simulink model "IC_Project"  (R2022b)
settings: Solver=FixedStepAuto  StartTime=0.0  StopTime=50  FixedStep=Ts  RelTol=1e-6
values from neighbouring files (symbols this model uses):
  g = 9.81    [aero_guid_dat.m]
  Iyy = 182.5/(Kg2slug*m2ft^2)    (= 247.436636441)    [aero_guid_dat.m]
  R = 287.26    [aero_guid_dat.m]
undefined symbols (not defined in the file or in its folder): AF, b_u, Delta_u, Delta_z_rotor, Dis, E_a, GE_flag, I_rotor, IC, inertia_u, Ixx, Izz, K1, K2, K3, K4, k_e, k_m, lambda, m, m_u, N_n, N_p, N_u, n_u, n_y, Out_sampleTime, phi_max, Q, R_eq, T_M, T_u, T_u_u, tau_m, theta_max, Ts
libraries: sharedtransform x1, sharedutil x1, simulink x1
settings Model: Creator=Mahdi  LastModifiedBy=Mahdi

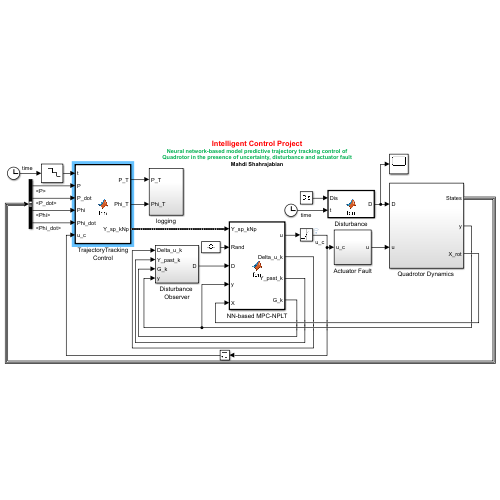
[thumbnail: Simulink's stored preview of the top-level diagram]
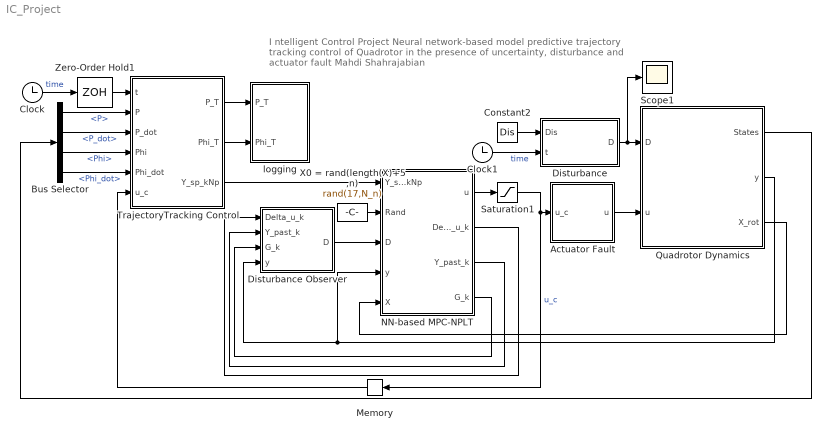
== system IC_Project ==
  note: I ntelligent Control Project
      | Neural network-based model predictive trajectory tracking control of Quadrotor in the presence of uncertainty, disturbance and actuator fault
      | Mahdi Shahrajabian
  Actuator Fault : Subsystem
  Bus Selector : BusSelector  OutputSignals=P,P_dot,Phi,Phi_dot
  Clock : Clock
  Clock1 : Clock
  Constant2 : Constant  Value=Dis
  Disturbance : MATLAB Function  TreatAsAtomicUnit=on
  Disturbance Observer : Subsystem
  Memory : Memory  InitialCondition=m*g*[1;1;1;1]/4
  NN-based MPC-NPLT : MATLAB Function  TreatAsAtomicUnit=on
  "Quadrotor Dynamics " : Subsystem  VariantControl=Choice_1
  Saturation1 : Saturate  UpperLimit=T_M  LowerLimit=0
  Scope1 : Scope
  TrajectoryTracking Control : MATLAB Function  TreatAsAtomicUnit=on
  X0 = rand(length(X)+5,n) : Constant  Value=rand(17,N_n)
  Zero-Order Hold1 : ZeroOrderHold  SampleTime=Ts
  logging : Subsystem
  wires:
  "Quadrotor Dynamics "/3(X_rot) -> NN-based MPC-NPLT/5(X)
  Zero-Order Hold1/1 -> TrajectoryTracking Control/1(t)
  Memory/1 -> TrajectoryTracking Control/6(u_c)
  "Quadrotor Dynamics "/1(States) -> Bus Selector/1
  Clock/1 -> Zero-Order Hold1/1  "time"
  Bus Selector/1 -> TrajectoryTracking Control/2(P)  "<P>"
  Bus Selector/2 -> TrajectoryTracking Control/3(P_dot)  "<P_dot>"
  Bus Selector/3 -> TrajectoryTracking Control/4(Phi)  "<Phi>"
  Bus Selector/4 -> TrajectoryTracking Control/5(Phi_dot)  "<Phi_dot>"
  TrajectoryTracking Control/3(Y_sp_kNp) -> NN-based MPC-NPLT/1(Y_sp_kNp)
  Disturbance/1(D) -> Scope1/1, "Quadrotor Dynamics "/1(D)
  TrajectoryTracking Control/2(Phi_T) -> logging/2(Phi_T)
  TrajectoryTracking Control/1(P_T) -> logging/1(P_T)
  X0 = rand(length(X)+5,n)/1 -> NN-based MPC-NPLT/2(Rand)
  "Quadrotor Dynamics "/2(y) -> NN-based MPC-NPLT/4(y), Disturbance Observer/4(y)
  Disturbance Observer/1(D) -> NN-based MPC-NPLT/3(D)
  NN-based MPC-NPLT/2(Delta_u_k) -> Disturbance Observer/1(Delta_u_k)
  NN-based MPC-NPLT/3(Y_past_k) -> Disturbance Observer/2(Y_past_k)
  NN-based MPC-NPLT/4(G_k) -> Disturbance Observer/3(G_k)
  Constant2/1 -> Disturbance/1(Dis)
  Actuator Fault/1(u) -> "Quadrotor Dynamics "/2(u)
  Clock1/1 -> Disturbance/2(t)  "time"
  NN-based MPC-NPLT/1(u) -> Saturation1/1
  Saturation1/1 -> Memory/1, Actuator Fault/1(u_c)  "u_c"

== system IC_Project/Actuator Fault ==
  u_c : Inport
  Actuator Fault1 : MATLAB Function  TreatAsAtomicUnit=on
  Clock : Clock
  Constant3 : Constant  Value=AF
  Scope : Scope
  Zero-Order Hold : ZeroOrderHold  SampleTime=Ts
  u : Outport
  wires:
  Zero-Order Hold/1 -> Actuator Fault1/2(u_c)
  Constant3/1 -> Actuator Fault1/1(AF)
  Clock/1 -> Actuator Fault1/3(t)
  Actuator Fault1/1(u) -> u/1
  u_c/1 -> Zero-Order Hold/1, Scope/1

== system IC_Project/Disturbance Observer ==
  Delta_u_k : Inport
  Y_past_k : Inport  Port=2
  G_k : Inport  Port=3
  y : Inport  Port=4
  MATLAB Function : MATLAB Function  TreatAsAtomicUnit=on
  Previous Steps : Subsystem
  Previous Steps1 : Subsystem
  Previous Steps2 : Subsystem
  D : Outport
  wires:
  MATLAB Function/1(D) -> D/1
  y/1 -> MATLAB Function/1(y)
  Delta_u_k/1 -> Previous Steps/1(Delta_u_k)
  Previous Steps/1(Delta_u_past) -> MATLAB Function/4(Delta_u_past)
  Previous Steps1/1(G_past) -> MATLAB Function/3(G_past)
  Previous Steps2/1(Y_past_past) -> MATLAB Function/2(Y_past_past)
  Y_past_k/1 -> Previous Steps2/1(Y_past_k)
  G_k/1 -> Previous Steps1/1(G_k)

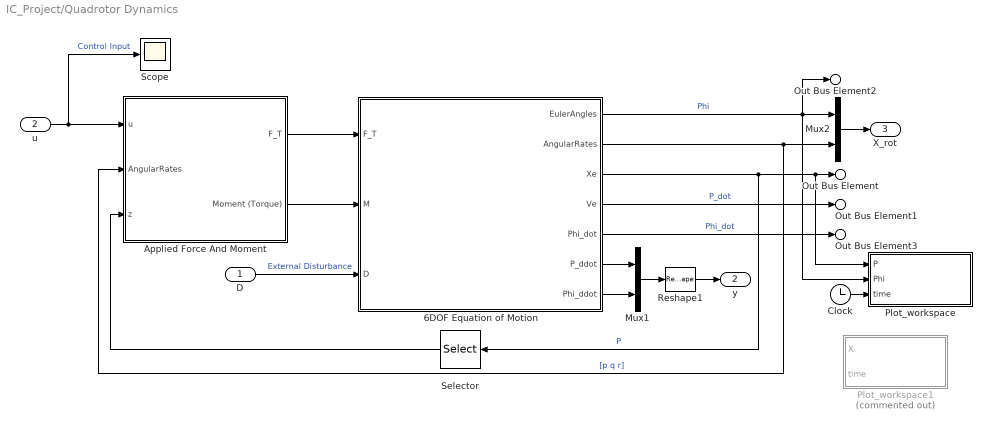
== system IC_Project/Quadrotor Dynamics  ==
  D : Inport
  u : Inport  Port=2
  6DOF Equation of Motion : Subsystem  mask{m=m_u, I=inertia_u, X0=IC.X, V0=IC.V, EA0=IC.EA, RR0=IC.AR}
      mask prompts: m "Quadrotor mass (m) - (kg):"; I "Quadrotor Moment of Inertia matrix (I) - (kg.m^2):"; X0 "Initial position in inertial axes [Xe, Ye, Ze] - (m):"; V0 "Initial velocity in body axes [u,v,w] - (m/s):"; EA0 "Initial Euler angles [roll, pitch, yaw] - (rad):"; RR0 "Initial body rotation rates [p,q,r] - (rad/s):"
      mask help: 6dof equations of motion of quadrotor
      mask DialogControl Container5 Prompt: Parameters
      mask DialogControl Container7 Prompt: Initial conditions
      mask Display: disp("6DOF Equation of motion\n(Euler Angles)")
  Applied Force And Moment : Subsystem  mask{T_u=T_u_u, b=b_u}
  Clock : Clock
  Mux1 : Mux  Inputs=2
  Mux2 : Mux  Inputs=2
  Plot_workspace : Subsystem
  Plot_workspace1 : Subsystem  Commented=on
  Reshape1 : Reshape  OutputDimensionality=Column vector (2-D)
  Scope : Scope
  Selector : Selector  InputPortWidth=3  IndexOptions=Index vector (dialog)  Indices=3  OutputSizes=1
  Out Bus Element : Outport  PortName=States  Element=P
  Out Bus Element1 : Outport  PortName=States  Element=P_dot
  Out Bus Element2 : Outport  PortName=States  Element=Phi
  Out Bus Element3 : Outport  PortName=States  Element=Phi_dot
  y : Outport  Port=2
  X_rot : Outport  Port=3
  wires:
  D/1 -> 6DOF Equation of Motion/3(D)  "External Disturbance"
  u/1 -> Scope/1, Applied Force And Moment/1(u)  "Control Input"
  Applied Force And Moment/2(Moment (Torque)) -> 6DOF Equation of Motion/2(M)
  6DOF Equation of Motion/2(AngularRates) -> Applied Force And Moment/2(AngularRates), Mux2/2  "[p q r]"
  Applied Force And Moment/1(F_T) -> 6DOF Equation of Motion/1(" F_T")
  6DOF Equation of Motion/4(Ve) -> Out Bus Element1/1  "P_dot"
  Selector/1 -> Applied Force And Moment/3(z)
  6DOF Equation of Motion/7(Phi_ddot) -> Mux1/2
  Reshape1/1 -> y/1
  Mux1/1 -> Reshape1/1
  6DOF Equation of Motion/6(P_ddot) -> Mux1/1
  Mux2/1 -> X_rot/1
  6DOF Equation of Motion/3(Xe) -> Selector/1, Plot_workspace/1(P), Out Bus Element/1  "P"
  6DOF Equation of Motion/1(EulerAngles) -> Out Bus Element2/1, Plot_workspace/2(Phi), Mux2/1  "Phi"
  6DOF Equation of Motion/5(Phi_dot) -> Out Bus Element3/1  "Phi_dot"
  Clock/1 -> Plot_workspace/3(time)

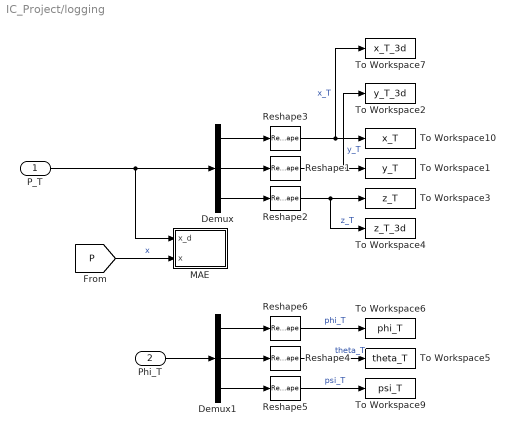
== system IC_Project/logging ==
  P_T : Inport
  Phi_T : Inport  Port=2
  Demux : Demux  Outputs=3
  Demux1 : Demux  Outputs=3
  MAE : Subsystem
  Reshape{1..6} (6 alike) : Reshape
  To Workspace1 : ToWorkspace  VariableName=y_T  SampleTime=Out_sampleTime
  To Workspace10 : ToWorkspace  VariableName=x_T  SampleTime=Out_sampleTime
  To Workspace2 : ToWorkspace  VariableName=y_T_3d  SampleTime=8*Out_sampleTime
  To Workspace3 : ToWorkspace  VariableName=z_T  SampleTime=Out_sampleTime
  To Workspace4 : ToWorkspace  VariableName=z_T_3d  SampleTime=8*Out_sampleTime
  To Workspace5 : ToWorkspace  VariableName=theta_T  SampleTime=Out_sampleTime
  To Workspace6 : ToWorkspace  VariableName=phi_T  SampleTime=Out_sampleTime
  To Workspace7 : ToWorkspace  VariableName=x_T_3d  SampleTime=8*Out_sampleTime
  To Workspace9 : ToWorkspace  VariableName=psi_T  SampleTime=Out_sampleTime
  wires:
  Reshape3/1 -> To Workspace7/1, To Workspace10/1  "x_T"
  Demux/1 -> Reshape3/1
  Demux/3 -> Reshape2/1
  Reshape2/1 -> To Workspace3/1, To Workspace4/1  "z_T"
  Reshape1/1 -> To Workspace2/1, To Workspace1/1  "y_T"
  Demux/2 -> Reshape1/1
  Reshape5/1 -> To Workspace9/1  "psi_T"
  Reshape4/1 -> To Workspace5/1  "theta_T"
  Demux1/2 -> Reshape4/1
  Demux1/1 -> Reshape6/1
  Demux1/3 -> Reshape5/1
  Reshape6/1 -> To Workspace6/1  "phi_T"
  Phi_T/1 -> Demux1/1
  P_T/1 -> Demux/1, MAE/1(x_d)
  [P] -> MAE/2(x)  "x"

== system IC_Project/Disturbance Observer/Previous Steps ==
  Delta_u_k : Inport
  Matrix Concatenate : Concatenate  NumInputs=10  ConcatenateDimension=2
  Reshape : Reshape  OutputDimensionality=Customize  OutputDimensions=[n_u 10]
  Unit Delay{,1..9} (10 alike) : UnitDelay  SampleTime=-1  HasFrameUpgradeWarning=on
  Delta_u_past : Outport
  wires:
  Matrix Concatenate/1 -> Reshape/1
  Delta_u_k/1 -> Unit Delay/1
  Unit Delay/1 -> Matrix Concatenate/1, Unit Delay1/1  "Delta_u_k1"
  Unit Delay1/1 -> Matrix Concatenate/2, Unit Delay2/1  "Delta_u_k2"
  Unit Delay2/1 -> Matrix Concatenate/3, Unit Delay3/1  "Delta_u_k3"
  Unit Delay3/1 -> Matrix Concatenate/4, Unit Delay4/1  "Delta_u_k4"
  Unit Delay4/1 -> Matrix Concatenate/5, Unit Delay5/1  "Delta_u_k5"
  Unit Delay5/1 -> Matrix Concatenate/6, Unit Delay6/1  "Delta_u_k6"
  Unit Delay6/1 -> Matrix Concatenate/7, Unit Delay7/1  "Delta_u_k7"
  Unit Delay7/1 -> Matrix Concatenate/8, Unit Delay8/1  "Delta_u_k8"
  Unit Delay8/1 -> Matrix Concatenate/9, Unit Delay9/1  "Delta_u_k9"
  Unit Delay9/1 -> Matrix Concatenate/10  "Delta_u_k10"
  Reshape/1 -> Delta_u_past/1

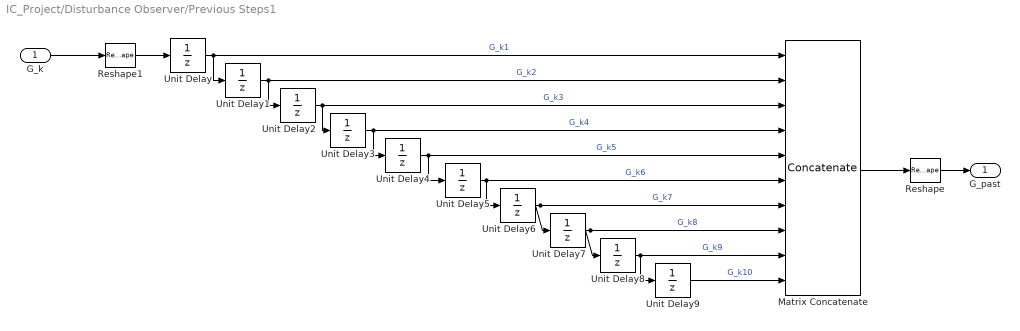
== system IC_Project/Disturbance Observer/Previous Steps1 ==
  G_k : Inport
  Matrix Concatenate : Concatenate  NumInputs=10  Mode=Multidimensional array  ConcatenateDimension=2
  Reshape : Reshape  OutputDimensionality=Customize  OutputDimensions=[60 24 10]
  Reshape1 : Reshape  OutputDimensionality=Customize  OutputDimensions=[60*24 1]
  Unit Delay{,1..9} (10 alike) : UnitDelay  SampleTime=-1  HasFrameUpgradeWarning=on
  G_past : Outport
  wires:
  Unit Delay9/1 -> Matrix Concatenate/10  "G_k10"
  Unit Delay8/1 -> Matrix Concatenate/9, Unit Delay9/1  "G_k9"
  Unit Delay7/1 -> Matrix Concatenate/8, Unit Delay8/1  "G_k8"
  Unit Delay6/1 -> Matrix Concatenate/7, Unit Delay7/1  "G_k7"
  Unit Delay5/1 -> Matrix Concatenate/6, Unit Delay6/1  "G_k6"
  Unit Delay4/1 -> Matrix Concatenate/5, Unit Delay5/1  "G_k5"
  Unit Delay3/1 -> Matrix Concatenate/4, Unit Delay4/1  "G_k4"
  Unit Delay2/1 -> Matrix Concatenate/3, Unit Delay3/1  "G_k3"
  Unit Delay1/1 -> Matrix Concatenate/2, Unit Delay2/1  "G_k2"
  Unit Delay/1 -> Matrix Concatenate/1, Unit Delay1/1  "G_k1"
  G_k/1 -> Reshape1/1
  Matrix Concatenate/1 -> Reshape/1
  Reshape/1 -> G_past/1
  Reshape1/1 -> Unit Delay/1

== system IC_Project/Disturbance Observer/Previous Steps2 ==
  Y_past_k : Inport
  Matrix Concatenate : Concatenate  NumInputs=10  Mode=Multidimensional array  ConcatenateDimension=2
  Reshape : Reshape  OutputDimensionality=Customize  OutputDimensions=[N_p*n_y 10]
  Unit Delay{,1..9} (10 alike) : UnitDelay  SampleTime=-1  HasFrameUpgradeWarning=on
  Y_past_past : Outport
  wires:
  Matrix Concatenate/1 -> Reshape/1
  Y_past_k/1 -> Unit Delay/1
  Unit Delay/1 -> Matrix Concatenate/1, Unit Delay1/1  "Y_past_k1"
  Unit Delay1/1 -> Matrix Concatenate/2, Unit Delay2/1  "Y_past_k2"
  Unit Delay2/1 -> Matrix Concatenate/3, Unit Delay3/1  "Y_past_k3"
  Unit Delay3/1 -> Matrix Concatenate/4, Unit Delay4/1  "Y_past_k4"
  Unit Delay4/1 -> Matrix Concatenate/5, Unit Delay5/1  "Y_past_k5"
  Unit Delay5/1 -> Matrix Concatenate/6, Unit Delay6/1  "Y_past_k6"
  Unit Delay6/1 -> Matrix Concatenate/7, Unit Delay7/1  "Y_past_k7"
  Unit Delay7/1 -> Matrix Concatenate/8, Unit Delay8/1  "Y_past_k8"
  Unit Delay8/1 -> Matrix Concatenate/9, Unit Delay9/1  "Y_past_k9"
  Unit Delay9/1 -> Matrix Concatenate/10  "Y_past_k10"
  Reshape/1 -> Y_past_past/1

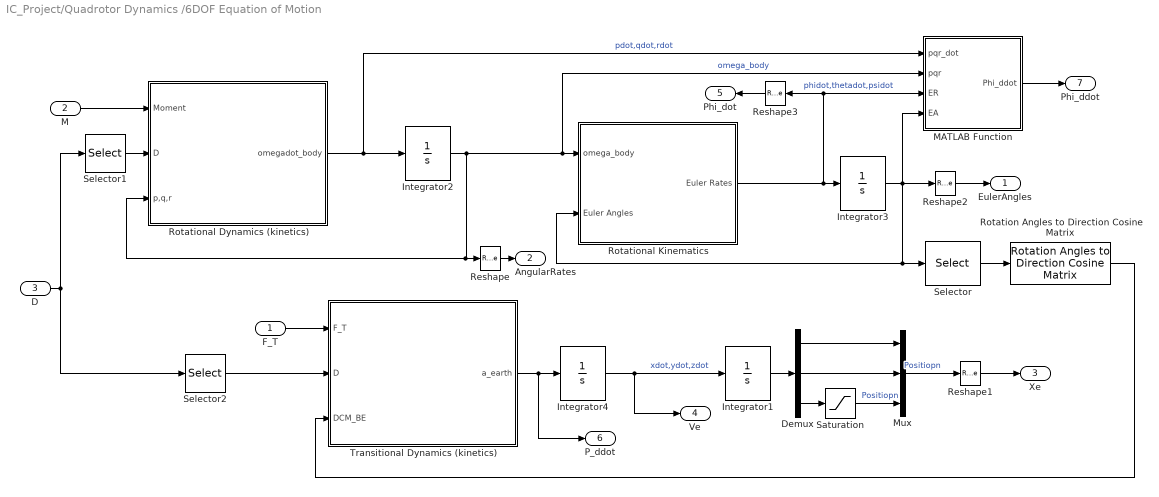
== system IC_Project/Quadrotor Dynamics /6DOF Equation of Motion ==
  " F_T" : Inport
  M : Inport  Port=2
  D : Inport  Port=3
  Demux : Demux  Outputs=3
  Integrator1 : Integrator  InitialCondition=X0
  Integrator2 : Integrator  InitialCondition=RR0
  Integrator3 : Integrator  InitialCondition=EA0  WrapState=on
  Integrator4 : Integrator  InitialCondition=V0
  MATLAB Function : MATLAB Function  TreatAsAtomicUnit=on
  Mux : Mux  Inputs=3
  Reshape{,1..3} (4 alike) : Reshape  OutputDimensionality=Column vector (2-D)
  Rotation Angles to Direction Cosine Matrix : sharedtransform/Rotation Angles to Direction Cosine Matrix  rotationOrder=ZYX  aMode=aMode
  Rotational Dynamics (kinetics) : Subsystem
  Rotational Kinematics : Subsystem
  Saturation : Saturate  UpperLimit=0  LowerLimit=-inf
  Selector : Selector  InputPortWidth=3  IndexOptions=Index vector (dialog)  Indices=[3 2 1]  OutputSizes=1
  Selector1 : Selector  InputPortWidth=6  IndexOptions=Index vector (dialog)  Indices=[1 2 3]  OutputSizes=1
  Selector2 : Selector  InputPortWidth=6  IndexOptions=Index vector (dialog)  Indices=[4 5 6]  OutputSizes=1
  Transitional Dynamics (kinetics) : Subsystem
  EulerAngles : Outport
  AngularRates : Outport  Port=2
  Xe : Outport  Port=3
  Ve : Outport  Port=4
  Phi_dot : Outport  Port=5
  P_ddot : Outport  Port=6
  Phi_ddot : Outport  Port=7
  wires:
  Mux/1 -> Reshape1/1  "Positiopn"
  M/1 -> Rotational Dynamics (kinetics)/1(Moment)
  " F_T"/1 -> Transitional Dynamics (kinetics)/1(" F_T")
  Rotational Kinematics/1(Euler Rates) -> Reshape3/1, MATLAB Function/3(ER), Integrator3/1  "phidot,thetadot,psidot"
  Integrator4/1 -> Ve/1, Integrator1/1  "xdot,ydot,zdot"
  Integrator2/1 -> MATLAB Function/2(pqr), Rotational Kinematics/1(omega_body), Reshape/1, Rotational Dynamics (kinetics)/3(p,q,r)  "omega_body"
  Selector/1 -> Rotation Angles to Direction Cosine Matrix/1
  Integrator3/1 -> MATLAB Function/4(EA), Selector/1, Rotational Kinematics/2(Euler Angles), Reshape2/1
  Rotation Angles to Direction Cosine Matrix/1 -> Transitional Dynamics (kinetics)/3(DCM_BE)
  Transitional Dynamics (kinetics)/1(a_earth) -> P_ddot/1, Integrator4/1
  D/1 -> Selector2/1, Selector1/1
  Selector1/1 -> Rotational Dynamics (kinetics)/2(D)
  Selector2/1 -> Transitional Dynamics (kinetics)/2(D)
  Integrator1/1 -> Demux/1
  Demux/1 -> Mux/1
  Demux/2 -> Mux/2
  Demux/3 -> Saturation/1
  Saturation/1 -> Mux/3  "Positiopn"
  MATLAB Function/1(Phi_ddot) -> Phi_ddot/1
  Rotational Dynamics (kinetics)/1(omegadot_body) -> MATLAB Function/1(pqr_dot), Integrator2/1  "pdot,qdot,rdot"
  Reshape2/1 -> EulerAngles/1
  Reshape1/1 -> Xe/1
  Reshape/1 -> AngularRates/1
  Reshape3/1 -> Phi_dot/1

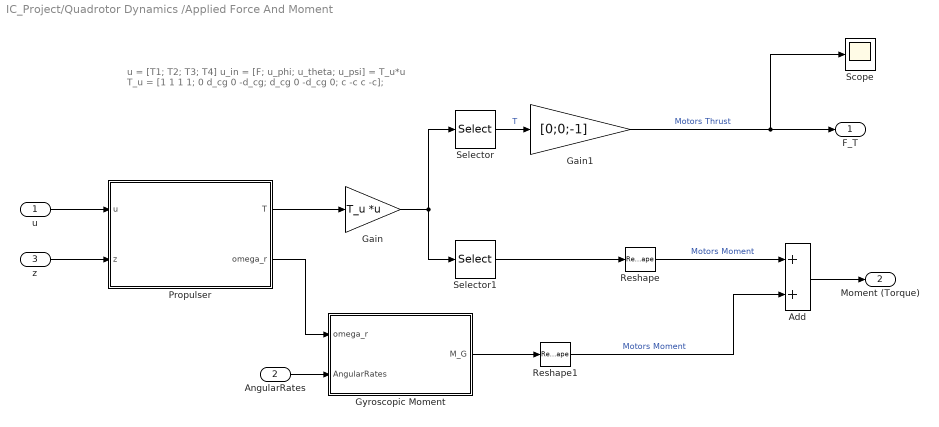
== system IC_Project/Quadrotor Dynamics /Applied Force And Moment ==
  note: u = [T1; T2; T3; T4]
      | u_in = [F; u_phi; u_theta; u_psi] = T_u*u
      | T_u = [1 1 1 1;
      |            0 d_cg 0 -d_cg;
      |           d_cg 0 -d_cg 0;
      |           c -c c -c];
  u : Inport
  AngularRates : Inport  Port=2
  z : Inport  Port=3
  Add : Sum
  Gain : Gain  Gain=T_u  Multiplication=Matrix(K*u)
  Gain1 : Gain  Gain=[0;0;-1]
  Gyroscopic Moment : Subsystem
  Propulser : Subsystem
  Reshape : Reshape  OutputDimensionality=Column vector (2-D)
  Reshape1 : Reshape  OutputDimensionality=Column vector (2-D)
  Scope : Scope
  Selector : Selector  InputPortWidth=4  IndexOptions=Index vector (dialog)  Indices=1  OutputSizes=1
  Selector1 : Selector  InputPortWidth=4  IndexOptions=Index vector (dialog)  Indices=[2 3 4]  OutputSizes=1
  F_T : Outport
  Moment (Torque) : Outport  Port=2
  wires:
  Gain1/1 -> Scope/1, F_T/1  "Motors Thrust"
  Gain/1 -> Selector/1, Selector1/1
  Propulser/1(T) -> Gain/1
  Selector1/1 -> Reshape/1
  u/1 -> Propulser/1(u)
  Selector/1 -> Gain1/1  "T"
  Add/1 -> Moment (Torque)/1
  Reshape/1 -> Add/1  "Motors Moment"
  Propulser/2(omega_r) -> Gyroscopic Moment/1(omega_r)
  AngularRates/1 -> Gyroscopic Moment/2(AngularRates)
  Gyroscopic Moment/1(M_G) -> Reshape1/1
  Reshape1/1 -> Add/2  "Motors Moment"
  z/1 -> Propulser/2(z)

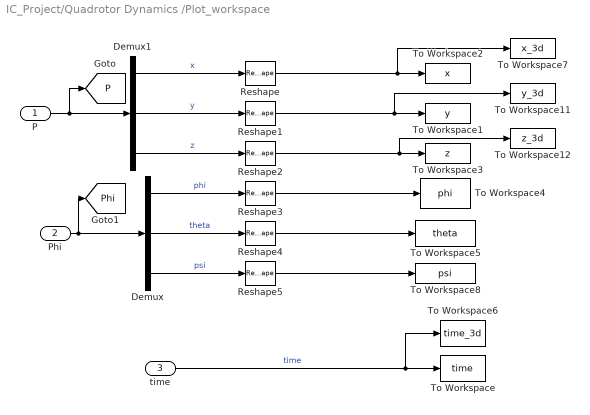
== system IC_Project/Quadrotor Dynamics /Plot_workspace ==
  P : Inport
  Phi : Inport  Port=2
  time : Inport  Port=3
  Demux : Demux  Outputs=3
  Demux1 : Demux  Outputs=3
  Reshape{,1..5} (6 alike) : Reshape
  To Workspace : ToWorkspace  VariableName=time  SampleTime=Out_sampleTime
  To Workspace1 : ToWorkspace  VariableName=y  SampleTime=Out_sampleTime
  To Workspace11 : ToWorkspace  VariableName=y_3d  SampleTime=8*Out_sampleTime
  To Workspace12 : ToWorkspace  VariableName=z_3d  SampleTime=8*Out_sampleTime
  To Workspace2 : ToWorkspace  VariableName=x  SampleTime=Out_sampleTime
  To Workspace3 : ToWorkspace  VariableName=z  SampleTime=Out_sampleTime
  To Workspace4 : ToWorkspace  VariableName=phi  SampleTime=Out_sampleTime
  To Workspace5 : ToWorkspace  VariableName=theta  SampleTime=Out_sampleTime
  To Workspace6 : ToWorkspace  VariableName=time_3d  SampleTime=8*Out_sampleTime
  To Workspace7 : ToWorkspace  VariableName=x_3d  SampleTime=8*Out_sampleTime
  To Workspace8 : ToWorkspace  VariableName=psi  SampleTime=Out_sampleTime
  tag scope: P=global, Phi=global
  wires:
  time/1 -> To Workspace6/1, To Workspace/1  "time"
  Reshape4/1 -> To Workspace5/1
  Reshape2/1 -> To Workspace3/1, To Workspace12/1
  Reshape5/1 -> To Workspace8/1
  Reshape/1 -> To Workspace2/1, To Workspace7/1
  Reshape1/1 -> To Workspace1/1, To Workspace11/1
  Reshape3/1 -> To Workspace4/1
  Demux/1 -> Reshape3/1  "phi"
  Demux/2 -> Reshape4/1  "theta"
  Demux/3 -> Reshape5/1  "psi"
  Phi/1 -> [Phi], Demux/1
  Demux1/1 -> Reshape/1  "x"
  Demux1/2 -> Reshape1/1  "y"
  Demux1/3 -> Reshape2/1  "z"
  P/1 -> Demux1/1, [P]

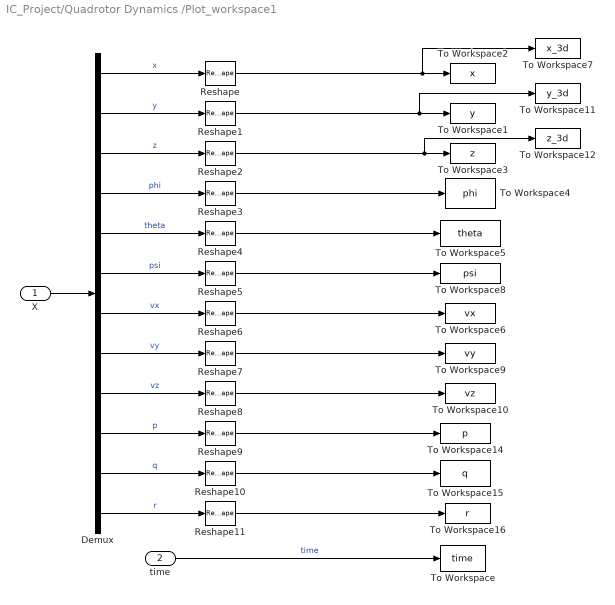
== system IC_Project/Quadrotor Dynamics /Plot_workspace1 ==
  X : Inport
  time : Inport  Port=2
  Demux : Demux  Outputs=12
  Reshape{,1..11} (12 alike) : Reshape
  To Workspace : ToWorkspace  VariableName=time  SampleTime=Out_sampleTime
      settings: Decimation=5
  To Workspace1 : ToWorkspace  VariableName=y  SampleTime=Out_sampleTime
      settings: Decimation=5
  To Workspace10 : ToWorkspace  VariableName=vz  SampleTime=Out_sampleTime
      settings: Decimation=5
  To Workspace11 : ToWorkspace  VariableName=y_3d  SampleTime=0.01
      settings: Decimation=20
  To Workspace12 : ToWorkspace  VariableName=z_3d  SampleTime=0.01
      settings: Decimation=20
  To Workspace14 : ToWorkspace  VariableName=p  SampleTime=Out_sampleTime
      settings: Decimation=5
  To Workspace15 : ToWorkspace  VariableName=q  SampleTime=Out_sampleTime
      settings: Decimation=5
  To Workspace16 : ToWorkspace  VariableName=r  SampleTime=Out_sampleTime
      settings: Decimation=5
  To Workspace2 : ToWorkspace  VariableName=x  SampleTime=Out_sampleTime
      settings: Decimation=5
  To Workspace3 : ToWorkspace  VariableName=z  SampleTime=Out_sampleTime
      settings: Decimation=5
  To Workspace4 : ToWorkspace  VariableName=phi  SampleTime=Out_sampleTime
      settings: Decimation=5
  To Workspace5 : ToWorkspace  VariableName=theta  SampleTime=Out_sampleTime
      settings: Decimation=5
  To Workspace6 : ToWorkspace  VariableName=vx  SampleTime=Out_sampleTime
      settings: Decimation=5
  To Workspace7 : ToWorkspace  VariableName=x_3d  SampleTime=0.01
      settings: Decimation=20
  To Workspace8 : ToWorkspace  VariableName=psi  SampleTime=Out_sampleTime
      settings: Decimation=5
  To Workspace9 : ToWorkspace  VariableName=vy  SampleTime=Out_sampleTime
      settings: Decimation=5
  wires:
  Demux/1 -> Reshape/1  "x"
  Demux/7 -> Reshape6/1  "vx"
  Demux/5 -> Reshape4/1  "theta"
  Demux/10 -> Reshape9/1  "p"
  Demux/9 -> Reshape8/1  "vz"
  Demux/11 -> Reshape10/1  "q"
  Demux/2 -> Reshape1/1  "y"
  Demux/3 -> Reshape2/1  "z"
  Demux/4 -> Reshape3/1  "phi"
  time/1 -> To Workspace/1  "time"
  Demux/8 -> Reshape7/1  "vy"
  Demux/6 -> Reshape5/1  "psi"
  Demux/12 -> Reshape11/1  "r"
  X/1 -> Demux/1
  Reshape/1 -> To Workspace7/1, To Workspace2/1
  Reshape1/1 -> To Workspace11/1, To Workspace1/1
  Reshape2/1 -> To Workspace12/1, To Workspace3/1
  Reshape3/1 -> To Workspace4/1
  Reshape4/1 -> To Workspace5/1
  Reshape5/1 -> To Workspace8/1
  Reshape6/1 -> To Workspace6/1
  Reshape7/1 -> To Workspace9/1
  Reshape8/1 -> To Workspace10/1
  Reshape9/1 -> To Workspace14/1
  Reshape10/1 -> To Workspace15/1
  Reshape11/1 -> To Workspace16/1

== system IC_Project/logging/MAE ==
  x_d : Inport
  x : Inport  Port=2
  Abs : Abs  SaturateOnIntegerOverflow=off
  Clock : Clock
  Display : Display
  Divide : Product  Inputs=*/
  IC : InitialCondition
  Integrator : Integrator
  Scope : Scope
  Subtract : Sum  Inputs=+-
  To Workspace : ToWorkspace  VariableName=MAE  SampleTime=-1
      settings: MaxDataPoints=1
  wires:
  x/1 -> Subtract/1
  x_d/1 -> Subtract/2
  Subtract/1 -> Abs/1
  Abs/1 -> Integrator/1
  Integrator/1 -> Divide/1
  Divide/1 -> Scope/1, Display/1, To Workspace/1  "MAE"
  Clock/1 -> IC/1
  IC/1 -> Divide/2

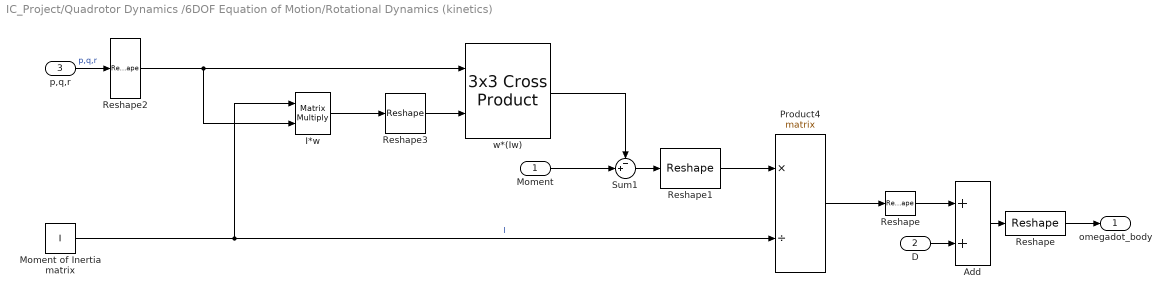
== system IC_Project/Quadrotor Dynamics /6DOF Equation of Motion/Rotational Dynamics (kinetics) ==
  Moment : Inport
  D : Inport  Port=2
  p,q,r : Inport  Port=3
  Add : Sum
  I*w : Product  Multiplication=Matrix(*)
  Moment of Inertia matrix : Constant  Value=I
  Product4 : Product  Inputs=*/  Multiplication=Matrix(*)  SaturateOnIntegerOverflow=on  OutDataTypeStr=Inherit: Same as first input
  Reshape : Reshape  OutputDimensionality=Column vector (2-D)
  "Reshape " : Reshape
  Reshape1 : Reshape  OutputDimensionality=Row vector (2-D)
  Reshape2 : Reshape  OutputDimensionality=Column vector (2-D)
  Reshape3 : Reshape
  Sum1 : Sum  Inputs=-+|  SaturateOnIntegerOverflow=on
  w*(Iw) : sharedutil/3x3 Cross Product  aMode=aMode
  omegadot_body : Outport
  wires:
  Reshape3/1 -> w*(Iw)/2
  I*w/1 -> Reshape3/1
  Reshape2/1 -> w*(Iw)/1, I*w/2
  p,q,r/1 -> Reshape2/1  "p,q,r"
  Moment/1 -> Sum1/2
  Sum1/1 -> Reshape1/1
  w*(Iw)/1 -> Sum1/1
  Moment of Inertia matrix/1 -> Product4/2, I*w/1  "I"
  Reshape1/1 -> Product4/1
  Product4/1 -> Reshape/1
  Add/1 -> "Reshape "/1
  D/1 -> Add/2
  "Reshape "/1 -> omegadot_body/1
  Reshape/1 -> Add/1

== system IC_Project/Quadrotor Dynamics /6DOF Equation of Motion/Rotational Kinematics ==
  omega_body : Inport
  Euler Angles : Inport  Port=2
  Mux1 : Mux  Inputs=[3 3 3]
  Mux2 : Mux  Inputs=3
  phidot : Fcn  Expr=u[1]+(u[2]*u[4]+u[3]*u[7])*(u[5]/u[8])
  psidot : Fcn  Expr=(u[2]*u[4]+u[3]*u[7])/u[8]
  sincos : Trigonometry  Operator=sincos
  thetadot : Fcn  Expr=u[2]*u[7]-u[3]*u[4]
  Euler Rates : Outport
  wires:
  Euler Angles/1 -> sincos/1  "phi, theta, psi"
  sincos/2 -> Mux1/3
  Mux1/1 -> psidot/1, phidot/1, thetadot/1
  omega_body/1 -> Mux1/1  "p, q, r"
  phidot/1 -> Mux2/1
  psidot/1 -> Mux2/3
  thetadot/1 -> Mux2/2
  sincos/1 -> Mux1/2
  Mux2/1 -> Euler Rates/1

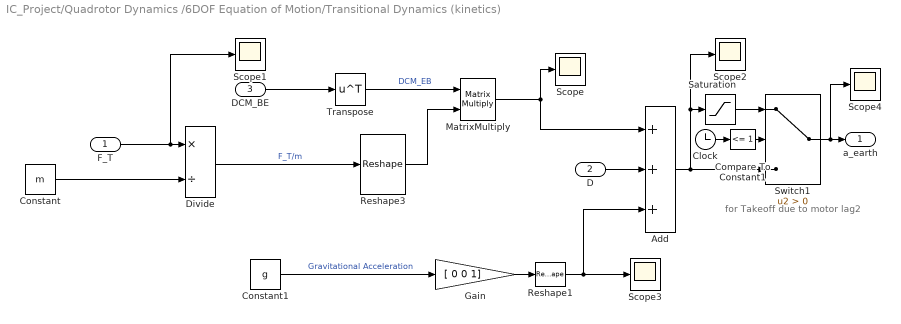
== system IC_Project/Quadrotor Dynamics /6DOF Equation of Motion/Transitional Dynamics (kinetics) ==
  note: for Takeoff due to motor lag2
  " F_T" : Inport
  D : Inport  Port=2
  DCM_BE : Inport  Port=3
  Add : Sum  Inputs=+++
  Clock : Clock
  Compare To Constant1 : simulink/Logic and Bit Operations/Compare To Constant  relop=<=  const=1  OutDataTypeStr=boolean
  Constant : Constant  Value=m
  Constant1 : Constant  Value=g
  Divide : Product  Inputs=*/
  Gain : Gain  Gain=[ 0 0 1]
  MatrixMultiply : Product  Multiplication=Matrix(*)
  Reshape1 : Reshape  OutputDimensionality=Column vector (2-D)
  Reshape3 : Reshape  OutputDimensionality=Column vector (2-D)
  Saturation : Saturate  UpperLimit=0  LowerLimit=-inf
  Scope{,1..4} (5 alike) : Scope
  Switch1 : Switch  Criteria=u2 > Threshold  SaturateOnIntegerOverflow=off  InputSameDT=off
  Transpose : Math  Operator=transpose
  a_earth : Outport
  wires:
  " F_T"/1 -> Scope1/1, Divide/1
  Constant/1 -> Divide/2
  Divide/1 -> Reshape3/1  "F_T/m"
  DCM_BE/1 -> Transpose/1
  Transpose/1 -> MatrixMultiply/1  "DCM_EB"
  Reshape3/1 -> MatrixMultiply/2
  Gain/1 -> Reshape1/1
  MatrixMultiply/1 -> Scope/1, Add/1
  Reshape1/1 -> Add/3, Scope3/1
  D/1 -> Add/2
  Constant1/1 -> Gain/1  "Gravitational Acceleration"
  Add/1 -> Switch1/3, Scope2/1, Saturation/1
  Saturation/1 -> Switch1/1
  Clock/1 -> Compare To Constant1/1
  Compare To Constant1/1 -> Switch1/2
  Switch1/1 -> Scope4/1, a_earth/1

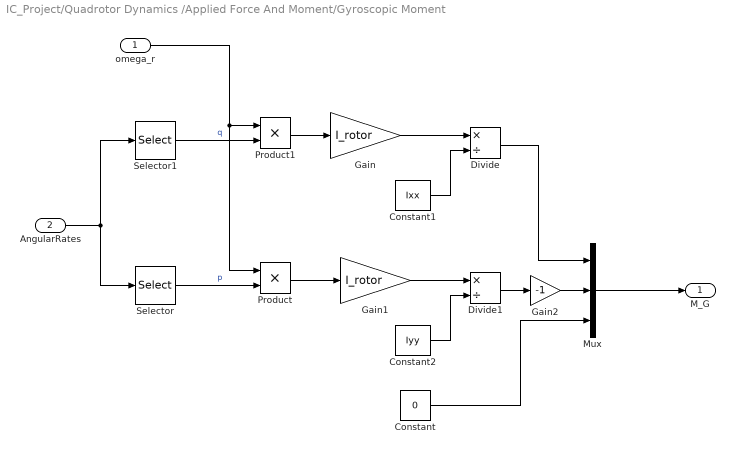
== system IC_Project/Quadrotor Dynamics /Applied Force And Moment/Gyroscopic Moment ==
  omega_r : Inport
  AngularRates : Inport  Port=2
  Constant : Constant  Value=0
  Constant1 : Constant  Value=Ixx
  Constant2 : Constant  Value=Iyy
  Divide : Product  Inputs=*/
  Divide1 : Product  Inputs=*/
  Gain : Gain  Gain=I_rotor
  Gain1 : Gain  Gain=I_rotor
  Gain2 : Gain  Gain=-1
  Mux : Mux  Inputs=3
  Product : Product
  Product1 : Product
  Selector : Selector  InputPortWidth=3  IndexOptions=Index vector (dialog)  Indices=1  OutputSizes=1
  Selector1 : Selector  InputPortWidth=3  IndexOptions=Index vector (dialog)  Indices=2  OutputSizes=1
  M_G : Outport
  wires:
  AngularRates/1 -> Selector/1, Selector1/1
  Selector/1 -> Product/2  "p"
  Selector1/1 -> Product1/2  "q"
  omega_r/1 -> Product1/1, Product/1
  Product1/1 -> Gain/1
  Product/1 -> Gain1/1
  Gain/1 -> Divide/1
  Constant1/1 -> Divide/2
  Gain1/1 -> Divide1/1
  Constant2/1 -> Divide1/2
  Divide/1 -> Mux/1
  Mux/1 -> M_G/1
  Divide1/1 -> Gain2/1
  Constant/1 -> Mux/3
  Gain2/1 -> Mux/2

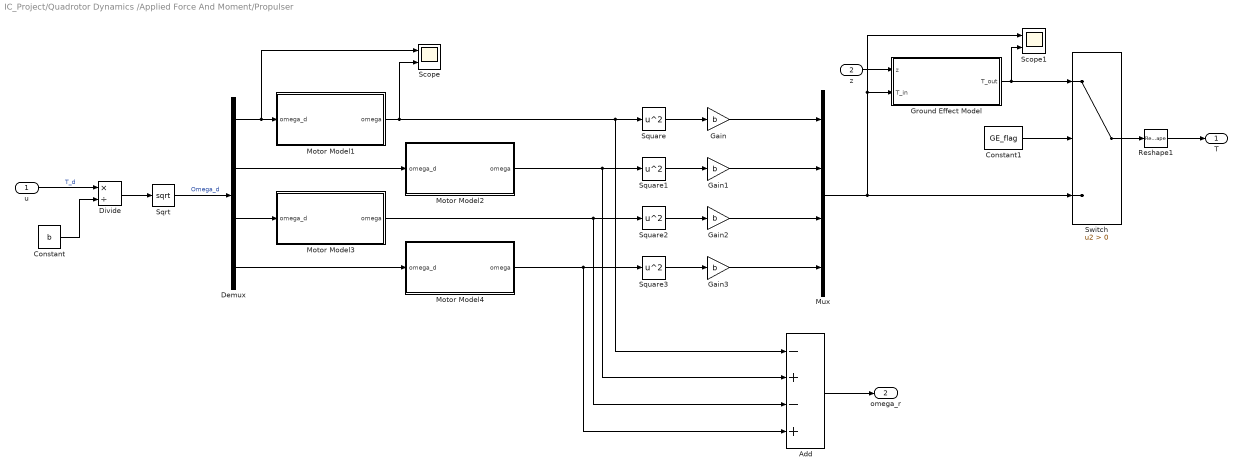
== system IC_Project/Quadrotor Dynamics /Applied Force And Moment/Propulser ==
  u : Inport
  z : Inport  Port=2
  Add : Sum  Inputs=-+-+
  Constant : Constant  Value=b
  Constant1 : Constant  Value=GE_flag
  Demux : Demux
  Divide : Product  Inputs=*/
  Gain{,1..3} (4 alike) : Gain  Gain=b
  Ground Effect Model : Subsystem
  Motor Model1 : Subsystem
  Motor Model2 : Subsystem
  Motor Model3 : Subsystem
  Motor Model4 : Subsystem
  Mux : Mux
  Reshape1 : Reshape  OutputDimensionality=Column vector (2-D)
  Scope : Scope  NumInputPorts=2
  Scope1 : Scope  NumInputPorts=2
  Sqrt : Sqrt
  Square{,1..3} (4 alike) : Math  Operator=square
  Switch : Switch  Criteria=u2 > Threshold  SaturateOnIntegerOverflow=off  InputSameDT=off
  T : Outport
  omega_r : Outport  Port=2
  wires:
  u/1 -> Divide/1  "T_d"
  Constant/1 -> Divide/2
  Sqrt/1 -> Demux/1  "Omega_d"
  Divide/1 -> Sqrt/1
  Demux/1 -> Scope/1, Motor Model1/1(omega_d)
  Demux/2 -> Motor Model2/1(omega_d)
  Demux/3 -> Motor Model3/1(omega_d)
  Demux/4 -> Motor Model4/1(omega_d)
  Square/1 -> Gain/1
  Square1/1 -> Gain1/1
  Square2/1 -> Gain2/1
  Square3/1 -> Gain3/1
  Motor Model2/1(omega) -> Add/2, Square1/1
  Motor Model3/1(omega) -> Add/3, Square2/1
  Motor Model4/1(omega) -> Add/4, Square3/1
  Gain3/1 -> Mux/4
  Gain/1 -> Mux/1
  Mux/1 -> Switch/3, Scope1/1, Ground Effect Model/2(T_in)
  Gain1/1 -> Mux/2
  Gain2/1 -> Mux/3
  Reshape1/1 -> T/1
  Switch/1 -> Reshape1/1
  Constant1/1 -> Switch/2
  Ground Effect Model/1(T_out) -> Scope1/2, Switch/1
  Add/1 -> omega_r/1
  Motor Model1/1(omega) -> Scope/2, Add/1, Square/1
  z/1 -> Ground Effect Model/1(z)

== system IC_Project/Quadrotor Dynamics /Applied Force And Moment/Propulser/Ground Effect Model ==
  note: Nobahari and Sharifi's Model
  z : Inport
  T_in : Inport  Port=2
  Add : Sum
  Add1 : Sum
  Constant : Constant  Value=R_eq
  Constant1 : Constant  Value=0.9926
  Constant2 : Constant  Value=-Delta_z_rotor
  Divide1 : Product  Inputs=*/
  Gain : Gain  Gain=0.03794
  Gain1 : Gain  Gain=2
  Product : Product
  Saturation : Saturate  UpperLimit=1.5  LowerLimit=1
  Square : Math  Operator=square
  T_out : Outport
  wires:
  z/1 -> Add1/1  "z"
  Constant1/1 -> Add/1
  Gain/1 -> Add/2
  Square/1 -> Gain/1
  Saturation/1 -> Product/1  "k_G"
  Divide1/1 -> Square/1
  Constant2/1 -> Add1/2
  Add1/1 -> Divide1/2  "z_rotor"
  Constant/1 -> Gain1/1
  Gain1/1 -> Divide1/1
  T_in/1 -> Product/2
  Product/1 -> T_out/1
  Add/1 -> Saturation/1

== system IC_Project/Quadrotor Dynamics /Applied Force And Moment/Propulser/Motor Model1 ==
  omega_d : Inport
  Gain : Gain  Gain=k_e
  Transfer Fcn1 : TransferFcn  Numerator=[k_m]  Denominator=[tau_m 1]
  omega : Outport
  wires:
  omega_d/1 -> Gain/1
  Gain/1 -> Transfer Fcn1/1  "v_d"
  Transfer Fcn1/1 -> omega/1

== system IC_Project/Quadrotor Dynamics /Applied Force And Moment/Propulser/Motor Model2 ==
  omega_d : Inport
  Gain : Gain  Gain=k_e
  Transfer Fcn1 : TransferFcn  Numerator=[k_m]  Denominator=[tau_m 1]
  omega : Outport
  wires:
  Transfer Fcn1/1 -> omega/1
  Gain/1 -> Transfer Fcn1/1  "v_d"
  omega_d/1 -> Gain/1

== system IC_Project/Quadrotor Dynamics /Applied Force And Moment/Propulser/Motor Model3 ==
  omega_d : Inport
  Gain : Gain  Gain=k_e
  Transfer Fcn1 : TransferFcn  Numerator=[k_m]  Denominator=[tau_m 1]
  omega : Outport
  wires:
  omega_d/1 -> Gain/1
  Gain/1 -> Transfer Fcn1/1  "v_d"
  Transfer Fcn1/1 -> omega/1

== system IC_Project/Quadrotor Dynamics /Applied Force And Moment/Propulser/Motor Model4 ==
  omega_d : Inport
  Gain : Gain  Gain=k_e
  Transfer Fcn1 : TransferFcn  Numerator=[k_m]  Denominator=[tau_m 1]
  omega : Outport
  wires:
  Transfer Fcn1/1 -> omega/1
  Gain/1 -> Transfer Fcn1/1  "v_d"
  omega_d/1 -> Gain/1

== matlab function IC_Project/TrajectoryTracking Control ==
  settings: updateMethod=DISCRETE  sampleTime=0.01
  data: P_T output size=[3 1]; Phi_T output size=[3 1]; Y_sp_kNp output size=[N_p*n_y,1]; t input; P input size=[3 1]; P_dot input size=[3 1]; Phi input size=[3 1]; Phi_dot input size=[3 1]; u_c input; Ts parameter; N_p parameter; n_y parameter; m parameter; E_a parameter; phi_max parameter; theta_max parameter; K1 parameter; K2 parameter; K3 parameter; K4 parameter
function [P_T,Phi_T,Y_sp_kNp] = fcn(t, P,P_dot,Phi,Phi_dot, u_c, Ts, N_p, n_y, m, E_a, phi_max, theta_max, K1, K2, K3, K4)
%% Persistent Variables
    persistent y_sp_i
        if isempty(y_sp_i)
            y_sp_i = zeros(n_y,1);
        end
    persistent Y_sp
        if isempty(Y_sp)
            Y_sp = zeros(N_p*n_y,1);
        end
    persistent phi_angle_T_k
        if isempty(phi_angle_T_k)
            phi_angle_T_k = 0;
        end
    persistent theta_angle_T_k
        if isempty(theta_angle_T_k)
            theta_angle_T_k = 0;
        end
    persistent PHI_T
        if isempty(PHI_T)
            PHI_T = zeros(3,N_p);
        end
%% Desired Trajectory
    % x_T = @(t) t;
    x_T = @(t) 5*sin(2*pi*t/10+pi/4);
    % y_T = @(t) 0;
    y_T = @(t) 8*cos(2*pi*t/15+pi/3);
    z_T = @(t) -2*t;
    P_T = [x_T(t);y_T(t);z_T(t)];
    % P_dot_T = @(t) [1;0;-2];
    P_dot_T = @(t) [pi*cos(2*pi*t/10+pi/4);-16*pi/15*sin(2*pi*t/15+pi/3);-2];
    P_ddot_T = @(t) [-2*pi^2/10*sin(2*pi*t/10+pi/4);-32*pi^2/15^2*cos(2*pi*t/15+pi/3);0];
    psi_T = @(t) 0;
    psi_dot_T = @(t) 0;

%% Future Output Set-point
    F = sum(u_c);
    % saturation
    if F<=5
        F = 5;
    elseif F>=30
        F = 30;
    end
    for i = 1:N_p
        P_ddot_sp = P_ddot_T(t+Ts)+K1*(P_dot_T(t+Ts)-P_dot)+K2*(P_T-P)+E_a.*sign(P_dot_T(t)-P_dot);
        phi_angle_T_k1 = - m*[sin(Phi(3)) -cos(Phi(3))]*[P_ddot_sp(1);P_ddot_sp(2)]/F;
        phi_angle_T_k1 = max(min(phi_angle_T_k1, 1), -1);
        phi_angle_T_k1 = asin(phi_angle_T_k1);
        theta_angle_T_k1 = (- m*[cos(Phi(3)) sin(Phi(3))]*[P_ddot_sp(1);P_ddot_sp(2)]/F)/cos(phi_angle_T_k1); 
        theta_angle_T_k1 = max(min(theta_angle_T_k1, 1), -1);
        theta_angle_T_k1 = asin(theta_angle_T_k1);
        % saturation
        if phi_angle_T_k1 >= phi_max
            phi_angle_T_k1 = phi_max;
        elseif phi_angle_T_k1 <= -phi_max
            phi_angle_T_k1 = -phi_max;
        end
        if theta_angle_T_k1 >= theta_max
            theta_angle_T_k1 = theta_max;
        elseif theta_angle_T_k1 <= -theta_max
            theta_angle_T_k1 = -theta_max;
        end
        Phi_TT = @(t)[phi_angle_T_k1;theta_angle_T_k1;psi_T(t)];
        PHI_T(:,i) = Phi_TT(t);
        Phi_dot_T = @(t)[(phi_angle_T_k1-phi_angle_T_k)/Ts;(theta_angle_T_k1-theta_angle_T_k)/Ts ;psi_dot_T(t)];
        Phi_ddot_sp = -K3*(Phi_dot-Phi_dot_T(t))-K4.*(Phi-Phi_TT(t));
        y_sp_i = [P_ddot_sp; Phi_ddot_sp];
        Y_sp(i*n_y-(n_y-1):n_y*i,1)=y_sp_i';
        phi_angle_T_k = phi_angle_T_k1;
        theta_angle_T_k = theta_angle_T_k1;
    end
    Y_sp_kNp = Y_sp;
    Phi_T = PHI_T(:,1);
end

== matlab function IC_Project/Quadrotor Dynamics /6DOF Equation of Motion/MATLAB Function ==
  data: pqr_dot input; pqr input; Phi_ddot output; ER input; EA input
function Phi_ddot = fcn(pqr_dot,pqr,ER,EA)

Phi_ddot = [pqr_dot(1)+pqr_dot(2)*sin(EA(1))*tan(EA(2))+pqr(2)*ER(1)*cos(EA(1))*tan(EA(2))+pqr(2)*ER(2)*sin(EA(1))*(1+tan(EA(2))^2)+...
            pqr_dot(3)*cos(EA(1))*tan(EA(2))-pqr(3)*ER(1)*sin(EA(1))*tan(EA(2))+pqr(3)*ER(2)*cos(EA(1))*(1+tan(EA(2))^2);
            pqr_dot(2)*cos(EA(1))-pqr(2)*ER(1)*sin(EA(1))-pqr_dot(3)*sin(EA(1))-pqr(3)*ER(1)*cos(EA(1));
            pqr_dot(2)*sin(EA(1))*sec(EA(2))+pqr(2)*ER(1)*cos(EA(1))*sec(EA(2))+pqr(2)*ER(2)*sin(EA(1))*sec(EA(2))*tan(EA(2))+...
            pqr_dot(3)*cos(EA(1))*sec(EA(2))-pqr(3)*ER(1)*sin(EA(1))*sec(EA(2))+pqr(3)*ER(2)*cos(EA(1))*sec(EA(2))*tan(EA(2))
              ];

== matlab function IC_Project/NN-based MPC-NPLT ==
  settings: updateMethod=DISCRETE
  data: Y_sp_kNp input; Rand input; D input; y input size=[6 1]; X input size=6; u output size=4; g parameter; Ixx parameter; Iyy parameter; Izz parameter; N_u parameter; N_p parameter; n_u parameter; n_y parameter; Delta_u parameter; T_u parameter; Q parameter; R parameter; m parameter; Ts parameter; lambda parameter; N_n parameter; Delta_u_k output size=[4 1]; Y_past_k output size=[60 1]; G_k output size=[60 24]
function [u,Delta_u_k,Y_past_k,G_k] = fcn(Y_sp_kNp,Rand,D, y,X, g, Ixx, Iyy, Izz, N_u, N_p, n_u, n_y, Delta_u, T_u, Q, R, m, Ts, lambda, N_n)
    persistent u0
    if isempty(u0)
        u0 = m*g*[1;1;1;1]/4; 
    end
    persistent Y_past_kNp
    if isempty(Y_past_kNp)
        Y_past_kNp = zeros(60,1);
    end
    persistent Y_p_u
    if isempty(Y_p_u)
        Y_p_u = zeros(60,4); 
    end
    persistent G
    if isempty(G)
        G = zeros(60,4*(5+1));
    end
    persistent Delta_past_kNp
    if isempty(Delta_past_kNp)
        Delta_past_kNp = zeros(60,1);
    end
    persistent Delta_p_u
    if isempty(Delta_p_u)
        Delta_p_u = zeros(60,4); 
    end
    persistent G_Delta
    if isempty(G_Delta)
        G_Delta = zeros(60,4*(5+1));
    end
    n = 10;
    X_0 = -8 + 16*Rand(1:n,:);
    sigma = 1.2 + 3*Rand(n+1,:);
    W0 = -1 + 2*Rand(n+2:n+7,:);
    persistent W
    if isempty(W)
        W = W0'; 
    end
    persistent P
    if isempty(P)
        P = 1000*eye(N_n);
    end
    persistent mu
    if isempty(mu)
        mu = zeros(N_n,1); 
    end

    % TimeStep
    X0_i = X;
    X0 = X;

%% Y_past and Delta_past
     w = W;
    for i = 1:N_p
        [X_p,y_past] = Dynamics(u0,X0,m,g,T_u,Ixx,Iyy,Izz,Ts);
        Y_past_kNp(i*n_y-(n_y-1):n_y*i,1)=y_past';
        % X_N = normalize([X0;u0]);
        X_N = [X0;u0];
        for j=1:N_n
            mu(j,1) = exp(-(X_N-X_0(:,j))'*(X_N-X_0(:,j))/(2*sigma(j)));
        end
        Delta_past = NN_Delta_predictor(w,mu);
        Delta_past_kNp(i*n_y-(n_y-1):n_y*i,1)= Delta_past;
        X0 = X_p;
    end
%% NLPT (Nonlinear Prediction and Linearization along the Trajectory)
    for j = 1:N_u+1
        for k=1:n_u
            X0 = X0_i;
            ui = u0;
            for i=1:N_p
                if i>=j
                    ui(k,1) = u0(k,1)+Delta_u;
                else
                    ui(k,1) = u0(k,1);
                end
                [~,y_p] = Dynamics(ui,X0,m,g,T_u,Ixx,Iyy,Izz,Ts);
                Y_p_u(i*n_y-(n_y-1):n_y*i,k)=y_p';
                % X_N = normalize([X0;ui]);
                X_N = [X0;ui];
                for s=1:N_n
                     mu(s,1) = exp(-(X_N-X_0(:,s))'*(X_N-X_0(:,s))/(2*sigma(s)));
                end
                Delta_p = NN_Delta_predictor(w,mu);
                Delta_p_u(i*n_y-(n_y-1):n_y*i,k)=Delta_p;
            end
        end
        G(1:n_y*N_p,n_u*j-(n_u-1):n_u*j)=(Y_p_u-[Y_past_kNp Y_past_kNp Y_past_kNp Y_past_kNp])/Delta_u;
        G_Delta(1:n_y*N_p,n_u*j-(n_u-1):n_u*j)=(Delta_p_u-[Delta_past_kNp Delta_past_kNp Delta_past_kNp Delta_past_kNp])/Delta_u;
    end
 %% MPC Optimizer
    % Delta_kNp = Delta_past_kNp+G_Delta*Delta_u_kNu;
    % Delta_u_kNu = (G'*Q*G+R)\(G'*Q*(Y_sp_kNp-Y_past_kNp-D));
    Delta_u_kNu = ((G+G_Delta)'*Q*(G+G_Delta)+R)\((G+G_Delta)'*Q*(Y_sp_kNp-Y_past_kNp-Delta_past_kNp-D));
    % Delta_u_kNu = (G'*Q*(G+G_Delta)+R)\(G'*Q*(Y_sp_kNp-Y_past_kNp-Delta_past_kNp));
    u = u0 +[eye(n_u,n_u) zeros(n_u,n_u*N_u)]*Delta_u_kNu;
    u0 = u;
%% Output for Disturbance Observer
    Y_past_k = Y_past_kNp;
    G_k = G;
    % Delta_u_k = [eye(n_u,n_u) zeros(n_u,n_u*N_u)]*Delta_u_kNu;
    Delta_u_k = [eye(4,4) zeros(4,4*5)]*Delta_u_kNu;

%% Update NN weights
    y_kNp = Y_past_kNp + Delta_past_kNp + (G+G_Delta) * Delta_u_kNu;
    % y_kNp = Y_past_kNp + Delta_past_kNp + G* Delta_u_kNu;
    y_n = [eye(n_y,n_y) zeros(n_y,n_y*(N_p-1))]*y_kNp;
    Delta = y-y_n;
    % X_N = normalize([X0_i;u0]);
    X_N = [X0;u0];
    for i=1:N_n
        mu(i,1) = exp(-(X_N-X_0(:,i))'*(X_N-X_0(:,i))/(2*sigma(i)));
    end
    Mu = mu;
    K = P*Mu/(lambda+Mu'*P*Mu);
    % K = P*Mu;
    P = (eye(N_n)-K*Mu')*P/lambda;
    e = Delta-W'*Mu;
    W = W + K*e';
    W = max(min(W, 10), -10);
    % w = W;
end

%% Discrete Equations of Quadrotor using the Runge-Kutta method
function [X_p_out,y_p_out] = Dynamics(u_in,X0_in,m,g,T_u,Ixx,Iyy,Izz,Ts)
    % X = [phi theta psi phi_dot theta_dot psi_dot]
    % u_in = [T1 T2 T3 T4]
    % u = [F, tau_phi tau_theta tau_psi]
    u_p = T_u*u_in;
    f = @(X,u) [X(4);
                X(5);
                X(6);
                (u(2)+X(5)*X(6)*(Iyy-Izz))/Ixx;
                (u(3)+X(4)*X(6)*(Izz-Ixx))/Iyy;    
                (u(4)+X(4)*X(5)*(Ixx-Iyy))/Izz];
    k1 = f(X0_in,u_p);
    k2 = f(X0_in+Ts*k1/2,u_p);
    k3 = f(X0_in+Ts*k2/2,u_p);
    k4 = f(X0_in+Ts*k3,u_p);
    X_p_out = X0_in+Ts*(k1+2*k2+2*k3+k4)/6;
    y_p_out = [-u_p(1)*(cos(X_p_out(3))*sin(X_p_out(2))*cos(X_p_out(1))+sin(X_p_out(3))*sin(X_p_out(1)))/m;
                -u_p(1)*(sin(X_p_out(3))*sin(X_p_out(2))*cos(X_p_out(1))-cos(X_p_out(3))*sin(X_p_out(1)))/m;
                g-u_p(1)*cos(X_p_out(1))*cos(X_p_out(2))/m;
                (u_p(2)+X_p_out(5)*X_p_out(6)*(Iyy-Izz))/Ixx;
                (u_p(3)+X_p_out(4)*X_p_out(6)*(Izz-Ixx))/Iyy;
                (u_p(4)+X_p_out(4)*X_p_out(5)*(Ixx-Iyy))/Izz];
end

function Delta_p = NN_Delta_predictor(w_in,Mu)
    Delta_p = w_in'*Mu;
end

== matlab function IC_Project/Disturbance Observer/MATLAB Function ==
  settings: updateMethod=DISCRETE
  data: y input double; D output size=[60 1]; Y_past_past input; G_past input; Delta_u_past input; N_p parameter; n_y parameter; n_u parameter; N_u parameter
function D = fcn(y,Y_past_past,G_past,Delta_u_past, N_p, n_y, n_u, N_u)
    persistent D1
    if isempty(D1)
        D1 = zeros(60,1); 
    end
    persistent gdu
    if isempty(D1)
        gdu = zeros(6,1) ;
    end
    for i=1:N_p
        y_past_k_i = Y_past_past((i-1)*n_y + 1:i*n_y,i);
        gdu = 0;
        for j=1:min(i,N_u+1)
            gdu = gdu + G_past((i-1)*n_y + 1:i*n_y, (j-1)*n_u + 1:j*n_u,i)*Delta_u_past(:,i-j+1);
        end
        y_k_i = y_past_k_i + gdu;
        D1(i*n_y-(n_y-1):n_y*i,1) = y - y_k_i;
    end
    D = D1;

== matlab function IC_Project/Actuator Fault/Actuator Fault1 ==
  data: AF input; u_c input; u output; t input
function u = fcn(AF,u_c, t)
if AF == 1
    if t<5
        u = u_c;
    elseif t>=5 && t<10
        u = diag([0.8,1,1,1])*u_c;
    elseif t>10 && t<15
        u = diag([0.8,0.7,1,1])*u_c;
    elseif t>15 && t<20
        u = diag([0.8,0.7,0.9,1])*u_c;
    else
        u = diag([0.8,0.7,0.9,0.9])*u_c;
    end
else
    u = u_c;
end

== matlab function IC_Project/Disturbance ==
  data: Dis input; D output; t input
function D = fcn(Dis, t)
if Dis == 1
    D = [0.05*sin(pi*t/2);
         0.05*sin(pi*t/3);
         0.02*cos(pi*t);
         0.1;
         0.1;
         0.1*sin(4*pi*t+pi/6)];
else
    D = zeros(6,1);
end
